simulink model "Stateflow_actionlineerror"  (R2015b)
settings: Solver=VariableStepAuto  StartTime=0.0  StopTime=10.0  RelTol=1e-3
settings Model: Creator=amyyang  LastModifiedBy=amyyang

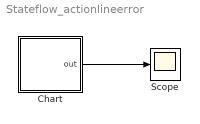
== system Stateflow_actionlineerror ==
  Chart : Stateflow chart  TreatAsAtomicUnit=on
  Scope : Scope
  wires:
  Chart/1(out) -> Scope/1

== stateflow chart Stateflow_actionlineerror/Chart ==
  state A
    en:
    out=0;
    state AA
      du:
      out++;
    state AB
      du:
      out--;
    (default) -> AA
  (default) -> A
  AA -> AB : [out > 10]
  data: out output double
